simulink model "BOOSTUJICOBA"  (R2023b)
settings: Solver=VariableStepAuto  StartTime=0.0  StopTime=20  RelTol=1e-3
undefined symbols (not defined in the file): Acid, Lead
libraries: spsSeriesRLCBranchLib x6, simulink x3, spsVoltageMeasurementLib x3, spsCurrentMeasurementLib x2, spsDiodeLib x2, spsMosfetLib x2, slpidlib x2, spsBatteryLib x1, spsGroundLib x1, spsPVArrayLib x1, spsPWMGeneratorDCDCLib x1, sps_lib x1
settings Model: Creator=M RAMANDA HIDAYAT  LastModifiedBy=M RAMANDA HIDAYAT

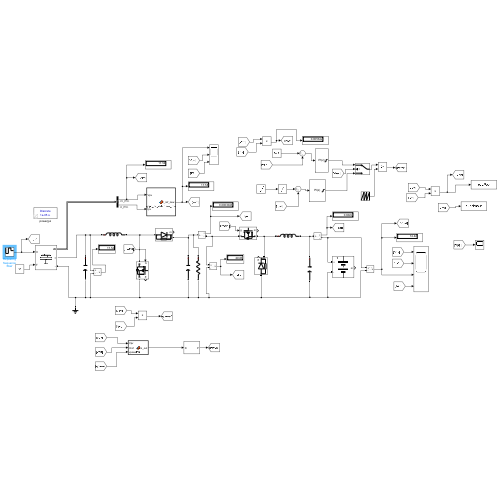
[thumbnail: Simulink's stored preview of the top-level diagram]
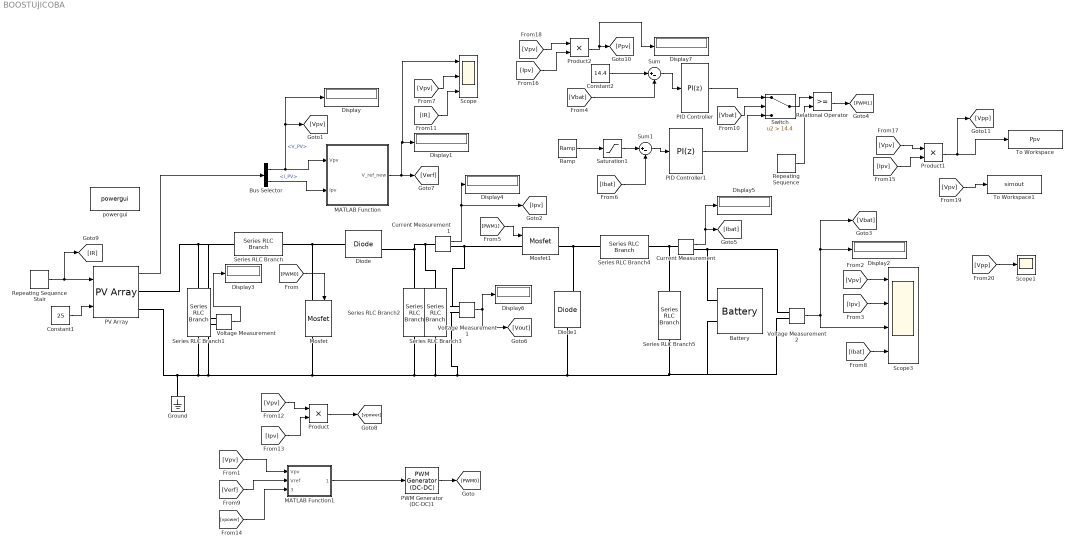
== system BOOSTUJICOBA ==
  Battery : spsBatteryLib/Battery  BatType=Lead-Acid  ShowTempParam=off  ThermalPreset=no  ShowAgeParam=off  NomV=12  NomQ=2  SOC=98.8  Batt_Tr=30  PresetModel=on  MaxQ=2.0833  MinV=9  FullV=13.0658  Dis_rate=0.4  R=0.06  Normal_OP=0.62056  expZone="[12.2171   0.00666667]"  current=[6.5 13 32.5]  Units=Time  Tci=20  NomT=20  T2=-30  MaxQ2=4.8  FullV2=7.1  Normal_OP2=5.655  expZone2="[6.58           1]"  Rca=0.6  ti=2000  Dp=0  Neq0=0  Tsim=1e6  Ta1=25  Qeol=5.4*0.9  Reol=0.013333*1.2  Char_age=[2.3478, 3]  Dis_age=[2.3478, 10]  N1=1500  N2=10500  N3=1000  N4=1400  Ta2=45  N5=950
  Bus Selector : BusSelector  OutputSignals=V_PV,I_PV
  Constant1 : Constant  Value=25
  Constant2 : Constant  Value=14.4
  Current Measurement : spsCurrentMeasurementLib/Current Measurement  PhasorSimulation=off  OutputType=Complex  PSBequivalent=0
  Current Measurement1 : spsCurrentMeasurementLib/Current Measurement  PhasorSimulation=off  OutputType=Complex  PSBequivalent=0
  Diode : spsDiodeLib/Diode  Ron=0.001  Lon=0  Vf=0.8  IC=0  UseSnubber=0  Rs=500  Cs=250e-9  Measurements=on
  Diode1 : spsDiodeLib/Diode  Ron=0.001  Lon=0  Vf=0.8  IC=0  UseSnubber=0  Rs=500  Cs=250e-9  Measurements=on
  Display{,1..7} (8 alike) : Display
  Ground : spsGroundLib/Ground  LConnTagsString=a
  MATLAB Function : MATLAB Function  TreatAsAtomicUnit=on  SystemSampleTime=1e-4
  MATLAB Function1 : MATLAB Function  TreatAsAtomicUnit=on
  Mosfet : spsMosfetLib/Mosfet  Ron=0.035  Lon=0  Rd=0.01  Vfd=1.3  IC=0  Rs=1e5  Cs=inf  Measurements=on
  Mosfet1 : spsMosfetLib/Mosfet  Ron=0.035  Lon=0  Rd=0.01  Vfd=1.3  IC=0  Rs=1e5  Cs=inf  Measurements=on
  PID Controller : slpidlib/PID Controller  Controller=PI  Form=Parallel  TimeDomain=Discrete-time  UseExternalTs=off  SampleTime=1e-05  IntegratorMethod=Forward Euler  FilterMethod=Forward Euler  ControllerParametersSource=internal  P=0.01  I=0.03  UseKiTs=off  D=0  N=100  UseFilter=on  TunerSelectOption=Transfer Function Based (PID Tuner App)  InitialConditionSource=internal  InitialConditionForIntegrator=0  InitialConditionForFilter=0  DifferentiatorICPrevScaledInput=0  ExternalReset=none  TrackingMode=off  Kt=1  LimitOutput=on  SatLimitsSource=internal  UpperSaturationLimit=1  LowerSaturationLimit=0  LinearizeAsGain=on  AntiWindupMode=none  Kb=1  LimitIntegrator=off  UpperIntegratorSaturationLimit=inf  LowerIntegratorSaturationLimit=-inf  POutMin=[]  POutMax=[]  IOutMin=[]  IOutMax=[]  DOutMin=[]  DOutMax=[]  NOutMin=[]  NOutMax=[]  SumOutMin=[]  SumOutMax=[]  SaturationOutMin=[]  SaturationOutMax=[]  PParamMin=[]  PParamMax=[]  IParamMin=[]  IParamMax=[]  DParamMin=[]  DParamMax=[]  NParamMin=[]  NParamMax=[]  KbParamMin=[]  KbParamMax=[]  KtParamMin=[]  KtParamMax=[]  KbOutMin=[]  KbOutMax=[]  KtOutMin=[]  KtOutMax=[]  IntegratorOutMin=[]  IntegratorOutMax=[]  FilterOutMin=[]  FilterOutMax=[]  SumI1OutMin=[]  SumI1OutMax=[]  SumI2OutMin=[]  SumI2OutMax=[]  SumI3OutMin=[]  SumI3OutMax=[]  SumI4OutMin=[]  SumI4OutMax=[]  SumDOutMin=[]  SumDOutMax=[]  DifferentiatorOutMin=[]  DifferentiatorOutMax=[]  FilterDiffOutCoefMin=[]  FilterDiffOutCoefMax=[]  ReciprocalOutMin=[]  ReciprocalOutMax=[]  SumDenOutMin=[]  SumDenOutMax=[]  SumNumOutMin=[]  SumNumOutMax=[]  DivideOutMin=[]  DivideOutMax=[]  UdiffTsProdOutMin=[]  UdiffTsProdOutMax=[]  NTsProdOutMin=[]  NTsProdOutMax=[]  UintegralTsProdOutMin=[]  UintegralTsProdOutMax=[]  UngainTsProdOutMin=[]  UngainTsProdOutMax=[]  ClampingZeroOutDataTypeStr=Inherit: Inherit via back propagation  ClampingZeroOutMin=[]  ClampingZeroOutMax=[]  FilterDenConstantOutDataTypeStr=Inherit: Inherit via back propagation  FilterDenConstantOutMin=[]  FilterDenConstantOutMax=[]  PCopyOutDataTypeStr=Inherit: Inherit via back propagation  PCopyOutMin=[]  PCopyOutMax=[]  NCopyOutDataTypeStr=Inherit: Inherit via back propagation  NCopyOutMin=[]  NCopyOutMax=[]  IntegratorContinuousStateAttributes=''  IntegratorStateMustResolveToSignalObject=off  IntegratorRTWStateStorageClass=Auto  FilterContinuousStateAttributes=''  FilterStateMustResolveToSignalObject=off  FilterRTWStateStorageClass=Auto  ParallelPVariant=InternalParameters  IdealPVariant=Disabled  IVariant=InternalParameters  DVariant=Disabled  IntegratorVariant=Discrete  SatVariant=Enabled  AWVariant=Passthrough  PCopyVariant=Disabled  TRVariant=Disabled  FdbkBlocksVariant=Forward  IdealPFdbkVariant=Disabled  SatFdbkVariant=Disabled  DerivativeFilterVariant=Disabled  NVariant=Disabled  NCopyVariant=Disabled_SignalSpec  FilterICVariant=Disabled  IntegratorICVariant=InternalICs  ExternalResetVariant=Disabled  TRSumVariant=Passthrough  SumFdbkVariant=Disabled  SumVariant=Sum_PI  TsampFilterVariant=InternalTs  TsampNgainVariant=Passthrough  TsampIntegralVariant=Disabled_SignalSpec  ExternalSaturationOutDataTypeStr=Inherit: Same as second input
  PID Controller1 : slpidlib/PID Controller  Controller=PI  Form=Parallel  TimeDomain=Discrete-time  UseExternalTs=off  SampleTime=1e-05  IntegratorMethod=Forward Euler  FilterMethod=Forward Euler  ControllerParametersSource=internal  P=1  I=1  UseKiTs=off  D=0  N=100  UseFilter=on  TunerSelectOption=Transfer Function Based (PID Tuner App)  InitialConditionSource=internal  InitialConditionForIntegrator=0  InitialConditionForFilter=0  DifferentiatorICPrevScaledInput=0  ExternalReset=none  TrackingMode=off  Kt=1  LimitOutput=on  SatLimitsSource=internal  UpperSaturationLimit=1  LowerSaturationLimit=0  LinearizeAsGain=on  AntiWindupMode=clamping  Kb=1  LimitIntegrator=off  UpperIntegratorSaturationLimit=inf  LowerIntegratorSaturationLimit=-inf  POutMin=[]  POutMax=[]  IOutMin=[]  IOutMax=[]  DOutMin=[]  DOutMax=[]  NOutMin=[]  NOutMax=[]  SumOutMin=[]  SumOutMax=[]  SaturationOutMin=[]  SaturationOutMax=[]  PParamMin=[]  PParamMax=[]  IParamMin=[]  IParamMax=[]  DParamMin=[]  DParamMax=[]  NParamMin=[]  NParamMax=[]  KbParamMin=[]  KbParamMax=[]  KtParamMin=[]  KtParamMax=[]  KbOutMin=[]  KbOutMax=[]  KtOutMin=[]  KtOutMax=[]  IntegratorOutMin=[]  IntegratorOutMax=[]  FilterOutMin=[]  FilterOutMax=[]  SumI1OutMin=[]  SumI1OutMax=[]  SumI2OutMin=[]  SumI2OutMax=[]  SumI3OutMin=[]  SumI3OutMax=[]  SumI4OutMin=[]  SumI4OutMax=[]  SumDOutMin=[]  SumDOutMax=[]  DifferentiatorOutMin=[]  DifferentiatorOutMax=[]  FilterDiffOutCoefMin=[]  FilterDiffOutCoefMax=[]  ReciprocalOutMin=[]  ReciprocalOutMax=[]  SumDenOutMin=[]  SumDenOutMax=[]  SumNumOutMin=[]  SumNumOutMax=[]  DivideOutMin=[]  DivideOutMax=[]  UdiffTsProdOutMin=[]  UdiffTsProdOutMax=[]  NTsProdOutMin=[]  NTsProdOutMax=[]  UintegralTsProdOutMin=[]  UintegralTsProdOutMax=[]  UngainTsProdOutMin=[]  UngainTsProdOutMax=[]  ClampingZeroOutDataTypeStr=Inherit: Inherit via back propagation  ClampingZeroOutMin=[]  ClampingZeroOutMax=[]  FilterDenConstantOutDataTypeStr=Inherit: Inherit via back propagation  FilterDenConstantOutMin=[]  FilterDenConstantOutMax=[]  PCopyOutDataTypeStr=Inherit: Inherit via back propagation  PCopyOutMin=[]  PCopyOutMax=[]  NCopyOutDataTypeStr=Inherit: Inherit via back propagation  NCopyOutMin=[]  NCopyOutMax=[]  IntegratorContinuousStateAttributes=''  IntegratorStateMustResolveToSignalObject=off  IntegratorRTWStateStorageClass=Auto  FilterContinuousStateAttributes=''  FilterStateMustResolveToSignalObject=off  FilterRTWStateStorageClass=Auto  ParallelPVariant=InternalParameters  IdealPVariant=Disabled  IVariant=InternalParameters  DVariant=Disabled  IntegratorVariant=Discrete  SatVariant=Enabled  AWVariant=DiscClampingParallel  PCopyVariant=Disabled  TRVariant=Disabled  FdbkBlocksVariant=Forward  IdealPFdbkVariant=Disabled  SatFdbkVariant=Disabled  DerivativeFilterVariant=Disabled  NVariant=Disabled  NCopyVariant=Disabled_SignalSpec  FilterICVariant=Disabled  IntegratorICVariant=InternalICs  ExternalResetVariant=Disabled  TRSumVariant=Passthrough  SumFdbkVariant=Disabled  SumVariant=Sum_PI  TsampFilterVariant=InternalTs  TsampNgainVariant=Passthrough  TsampIntegralVariant=Disabled_SignalSpec  ExternalSaturationOutDataTypeStr=Inherit: Same as second input
  PV Array : spsPVArrayLib/PV Array  Npar=1  Nser=1  PlotType=array @ 25 deg.C & specified irradiances  S_vec=[25]  Temp_C_vec="[  ]"  ModuleName=User-defined  PlotWhenSelected=off  Pm=50.052  Ncell=36  Voc=21.6  Isc=3.23  Vm=17.2  Im=2.91  beta_Voc_pc=-0.36099  alpha_Isc_pc=0.102  beta_Voc=-0.077974  alpha_Isc=0.0032946  IL=3.2481  I0=1.1906e-10  nI=0.97446  Rsh=107.2163  Rs=0.60203  RobustModel=off  RobustCellTemperature=313.3991  BAL=on  Tc=1e-6  Tfilter=5e-5
  PWM Generator (DC-DC)1 : spsPWMGeneratorDCDCLib/PWM Generator (DC-DC)  Fsw=5000  Ts=0
  Product : Product
  Product1 : Product
  Product2 : Product
  Ramp : simulink/Sources/Ramp  slope=0.5  start=0.5  InitialOutput=0
  Relational Operator : RelationalOperator  OutDataTypeStr=boolean  RndMeth=Simplest  InputSameDT=off
  Repeating Sequence : simulink/Sources/Repeating Sequence  rep_seq_t=[0 1/25000]  rep_seq_y=[0 1]
  Repeating Sequence Stair : simulink/Sources/Repeating Sequence Stair  OutValues=[400 800 600].'  tsamp=5  OutMin=[]  OutMax=[]  OutDataTypeStr=double  OutputDataTypeScalingMode=double  OutDataType=fixdt(0,8)  ConRadixGroup=Best Precision: Vector-wise  OutScaling=2^-12
  Saturation1 : Saturate  UpperLimit=1.5  LowerLimit=0
  Scope : Scope  NumInputPorts=3
  Scope1 : Scope
  Scope3 : Scope  NumInputPorts=4
  Series RLC Branch : spsSeriesRLCBranchLib/Series RLC Branch  LConnTagsString=__new0  RConnTagsString=__new0  BranchType=L  Resistance=1  Inductance=220e-6  SetiL0=off  InitialCurrent=0  Capacitance=1e-6  Setx0=off  InitialVoltage=0  Measurements=None
  Series RLC Branch1 : spsSeriesRLCBranchLib/Series RLC Branch  LConnTagsString=__new0  RConnTagsString=__new0  BranchType=C  Resistance=1  Inductance=42e-6  SetiL0=off  InitialCurrent=0  Capacitance=2200e-6  Setx0=off  InitialVoltage=0  Measurements=None
  Series RLC Branch2 : spsSeriesRLCBranchLib/Series RLC Branch  LConnTagsString=__new0  RConnTagsString=__new0  BranchType=C  Resistance=11.52  Inductance=42e-6  SetiL0=off  InitialCurrent=0  Capacitance=1000e-6  Setx0=on  InitialVoltage=24  Measurements=None
  Series RLC Branch3 : spsSeriesRLCBranchLib/Series RLC Branch  LConnTagsString=__new0  RConnTagsString=__new0  BranchType=R  Resistance=100  Inductance=42e-6  SetiL0=off  InitialCurrent=0  Capacitance=1000e-6  Setx0=on  InitialVoltage=24  Measurements=None
  Series RLC Branch4 : spsSeriesRLCBranchLib/Series RLC Branch  LConnTagsString=__new0  RConnTagsString=__new0  BranchType=L  Resistance=1  Inductance=750e-6  SetiL0=off  InitialCurrent=0  Capacitance=1e-6  Setx0=off  InitialVoltage=0  Measurements=None
  Series RLC Branch5 : spsSeriesRLCBranchLib/Series RLC Branch  LConnTagsString=__new0  RConnTagsString=__new0  BranchType=C  Resistance=11.52  Inductance=42e-6  SetiL0=off  InitialCurrent=0  Capacitance=2200e-6  Setx0=off  InitialVoltage=0  Measurements=None
  Sum : Sum  Inputs=|+-
  Sum1 : Sum  Inputs=|+-
  Switch : Switch  Criteria=u2 > Threshold  Threshold=14.4  SaturateOnIntegerOverflow=off  InputSameDT=off
  To Workspace : ToWorkspace  VariableName=Ppv  SaveFormat=Timeseries  SampleTime=1e-05
  To Workspace1 : ToWorkspace  VariableName=simout  SaveFormat=Timeseries  SampleTime=1e-05
  Voltage Measurement : spsVoltageMeasurementLib/Voltage Measurement  PhasorSimulation=off  OutputType=Complex  PSBequivalent=0
  Voltage Measurement1 : spsVoltageMeasurementLib/Voltage Measurement  PhasorSimulation=off  OutputType=Complex  PSBequivalent=0
  Voltage Measurement2 : spsVoltageMeasurementLib/Voltage Measurement  PhasorSimulation=off  OutputType=Complex  PSBequivalent=0
  powergui : sps_lib/powergui  Priority=1  SimulationMode=Discrete  SampleTime=1e-5  frequency=60  Iterations=50  frequencyindice=0  Pbase=100e6  ErrMax=1e-4  UnitsV=kV  UnitsW=MW  buscounter=0  FunctionMessages=off  echomessages=off  EnableUseOfTLC=off  CurrentSourceSwitches=off  DisableSnubberDevices=off  DisableRonSwitches=off  DisableVfSwitches=off  DisplayEquations=off  AutomaticDiscreteSolvers=off  SolverType=Tustin/Backward Euler (TBE)  Interpol=off  ExternalGateDelay=off  methode=off  Ts=100  x0status=blocks  SPID=on  SwTol=0  HookPort=off  NonlinearTolerance=1e-4  nMaxIteration=100  ContinueOnMaxIteration=off  RestoreLinks=warning  ResistiveCurrentMeasurement=off  Frange=[0:2:500]  Ylog=off  Xlog=on  ShowGrid=off  save=off  variable=ZData  structure=0  ZoomFFT=off  StartTime=0.0  cycles=1  DisplayStyle=1  fundamental=60  FreqAxis=off  MaxFrequency=1000  frequencyindicesteady=1  RmsSteady=1  display=off
  wires:
  Constant1/1 -> PV Array/2
  Voltage Measurement/1 -> Display3/1
  Voltage Measurement2/1 -> Scope3/3, [Vbat], Display2/1
  Current Measurement1/1 -> Display4/1, [Ipv]
  PV Array/1 -> Bus Selector/1
  [PWM0] -> Mosfet/1
  Bus Selector/1 -> Display/1, [Vpv], MATLAB Function/1(Vpv)  "<V_PV>"
  Bus Selector/2 -> MATLAB Function/2(Ipv)  "<I_PV>"
  MATLAB Function/1(V_ref_new) -> [Verf], Scope/1, Display1/1
  [Vpv] -> Scope3/1
  [Vbat] -> Sum/2
  Constant2/1 -> Sum/1
  Sum/1 -> PID Controller/1
  Repeating Sequence/1 -> Relational Operator/2
  Relational Operator/1 -> [PWM1]
  [PWM1] -> Mosfet1/1
  Current Measurement/1 -> Display5/1, [Ibat]
  [Ibat] -> Sum1/2
  Sum1/1 -> PID Controller1/1
  [Ibat] -> Scope3/4
  [Ipv] -> Scope3/2
  Saturation1/1 -> Sum1/1
  Ramp/1 -> Saturation1/1
  Voltage Measurement1/1 -> [Vout], Display6/1
  [Vpv] -> Scope/2
  PWM Generator (DC-DC)1/1 -> [PWM0]
  [IR] -> Scope/3
  [Vpv] -> MATLAB Function1/1(Vpv)
  [Verf] -> MATLAB Function1/2(Vref)
  [Vpv] -> Product/1
  [Ipv] -> Product/2
  Product/1 -> [vpower]
  [vpower] -> MATLAB Function1/3(vpower)
  MATLAB Function1/1(pwm_out) -> PWM Generator (DC-DC)1/1
  PID Controller/1 -> Switch/1
  Switch/1 -> Relational Operator/1
  [Vbat] -> Switch/2
  PID Controller1/1 -> Switch/3
  [Vpv] -> Product1/1
  [Ipv] -> Product1/2
  Product1/1 -> [Vpp], To Workspace/1
  [Ipv] -> Product2/2
  [Vpv] -> Product2/1
  Product2/1 -> Display7/1, [Ppv]
  [Vpv] -> To Workspace1/1
  Repeating Sequence Stair/1 -> PV Array/1, [IR]
  [Vpp] -> Scope1/1
  connections:
  Series RLC Branch1/LConn1 -- Voltage Measurement/LConn1 -- Series RLC Branch/LConn1 -- PV Array/RConn1
  Series RLC Branch/RConn1 -- Diode/LConn1 -- Mosfet/LConn1
  PV Array/RConn2 -- Ground/LConn1 -- Series RLC Branch1/RConn1 -- Voltage Measurement/LConn2 -- Mosfet/RConn1 -- Series RLC Branch3/RConn1 -- Voltage Measurement2/LConn2 -- Battery/LConn2 -- Series RLC Branch5/RConn1 -- Diode1/LConn1 -- Voltage Measurement1/LConn2 -- Series RLC Branch2/RConn1
  Mosfet1/LConn1 -- Voltage Measurement1/LConn1 -- Current Measurement1/RConn1
  Current Measurement1/LConn1 -- Series RLC Branch3/LConn1 -- Diode/RConn1 -- Series RLC Branch2/LConn1
  Series RLC Branch4/LConn1 -- Diode1/RConn1 -- Mosfet1/RConn1
  Series RLC Branch5/LConn1 -- Current Measurement/LConn1 -- Series RLC Branch4/RConn1
  Current Measurement/RConn1 -- Battery/LConn1 -- Voltage Measurement2/LConn1

== matlab function BOOSTUJICOBA/MATLAB Function ==
  data: Vpv input; V_ref_new output; Ipv input
function V_ref_new = mppt_po_adaptive_test(Vpv, Ipv)
% =========================================================================
% MPPT P&O ADAPTIVE - OPTIMIZED VERSION
% Status: Reduksi osilasi dan stabilitas steady-state
% =========================================================================
persistent V_ref_old P_old Vpv_old step_count initialization_done

% ---------- 1. SETUP PARAMETER ----------
V_max       = 21.0;     
V_min       = 13.5;     
update_step = 50;       % Memberi waktu hardware untuk stabil sebelum update
Step_Min    = 0.01;     % Langkah terkecil untuk presisi di puncak
Step_Max    = 0.01;     % Batasan agar tidak loncat drastis saat iradiasi berubah

% ---------- 2. INISIALISASI ----------
if isempty(initialization_done)
    V_ref_old = 17.0;   
    P_old     = 0; 
    Vpv_old   = 0;      
    step_count = 0;
    initialization_done = 1;
end

% ---------- 3. DELAY / SAMPLING RATE ----------
step_count = step_count + 1;
if step_count < update_step
    V_ref_new = V_ref_old;
    return;
end
step_count = 0; 

% ---------- 4. HITUNG PERUBAHAN ----------
P_new = Vpv * Ipv;
dP    = P_new - P_old;
dV    = Vpv - Vpv_old;

% ---------- 5. LOGIKA VARIABLE STEP (ADAPTIVE) ----------
Scaling_Factor = 0.02; % Diturunkan dari 0.1 untuk menghilangkan noise
Step_Size = abs(dP) * Scaling_Factor;

if Step_Size < Step_Min
    Step_Size = Step_Min;
elseif Step_Size > Step_Max
    Step_Size = Step_Max;
end

% ---------- 6. LOGIKA P&O DENGAN DEADBAND ----------
if abs(dP) < 0.15 % Zona mati diperlebar agar garis lurus saat stabil
    V_ref_new = V_ref_old;
else
    if dP > 0
        if dV > 0, V_ref_new = V_ref_old + Step_Size; 
        else,      V_ref_new = V_ref_old - Step_Size; end
    else
        if dV > 0, V_ref_new = V_ref_old - Step_Size; 
        else,      V_ref_new = V_ref_old + Step_Size; end
    end
end

% ---------- 7. SAFETY LIMITS & UPDATE ----------
if V_ref_new > V_max, V_ref_new = V_max;
elseif V_ref_new < V_min, V_ref_new = V_min; end

P_old = P_new; Vpv_old = Vpv; V_ref_old = V_ref_new;

== matlab function BOOSTUJICOBA/MATLAB Function1 ==
  data: Vpv input; pwm_out output; Vref input; vpower input
function pwm_out = fcn(Vpv, Vref, vpower)
% ====================================================
% SMC CONTROLLER FOR BOOST CONVERTER - STABLE VERSION
% ====================================================
persistent duty_cycle
if isempty(duty_cycle), duty_cycle = 0.5; end

% --- 1. HITUNG ERROR ---
error = Vpv - Vref;

% --- 2. ADAPTIVE GAIN (Dihaluskan untuk SMC) ---
% Nilai K diperkecil agar tidak terjadi chattering (getaran frekuensi tinggi)
if vpower > 100
    K = 0.001; 
elseif vpower > 60
    K = 0.0008; 
else
    K = 0.0005; 
end

% --- 3. LOGIKA PENGENDALI (RELAY-LIKE SMC) ---
% Jika Vpv > Vref, tambah duty cycle (sedot arus) untuk turunkan tegangan
% Jika Vpv < Vref, kurangi duty cycle untuk naikkan tegangan
deadband = 0.2; % Batas toleransi agar tidak bergetar di titik target

if error > deadband
    duty_cycle = duty_cycle + K;
elseif error < -deadband
    duty_cycle = duty_cycle - K;
end

% --- 4. SAFETY LIMITER ---
if duty_cycle > 0.95, duty_cycle = 0.95;
elseif duty_cycle < 0.05, duty_cycle = 0.05; end

pwm_out = duty_cycle;
